simulink model "boithitiko"  (Simulink 5.0)
settings: Solver=FixedStepDiscrete  StartTime=0.0  StopTime=inf  RelTol=1e-3
libraries: dspquant2 x1, dspbuff3 x1
CloseFcn:
  | rtwprivate ssgencode ModelCloseRequest boithitiko
settings Model: LastModifiedBy=efst  RTWOptions="-aEnforceIntegerDowncast=1 -aExtMode=0 -aExtModeTesting=0 -aFoldNonRolledExpr=1 -aForceParamTrailComments=0 -aGenerateComments=1 -aGenerateReport=0 -aIgnoreCustomStorageClasses=1 -aIncDataTypeInIds=0 -aIncHierarchyInIds=0 -aInlineInvariantSignals=0 -aInlinedPrmAccess=\"Literals\" -aLocalBlockOutputs=1 -aLogVarNameModifier=\"rt_\" -aMaxRTWIdLen=31 -aPrefixModelToSubsysFcnNames=1 -aRTWVerbose=1 -aRollThreshold=5 -aShowEliminatedStatements=0"

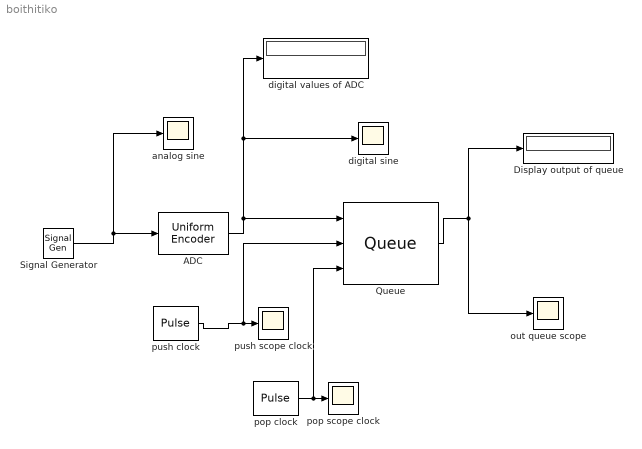
== system boithitiko ==
  ADC : dspquant2/Uniform Encoder  peak=1  bits=8  otype=Unsigned integer
  Display output of queue : Display
  Queue : dspbuff3/Queue  depth=3  trigger=Rising edge  overflow=Dynamic reallocation  pes=Warning  eso=off  fso=off  nso=off  clr=off  clrOutport=off
  Signal Generator : SignalGenerator  Frequency=1000
  analog sine : Scope
      settings: YMin=-1  YMax=1
  digital sine : Scope
      settings: TimeRange=0.001  YMin=0  YMax=275
  digital values of ADC : Display
  out queue scope : Scope
      settings: TimeRange=0.01  YMin=0  YMax=275  SaveName=ScopeData5
  "pop clock " : DiscretePulseGenerator  PulseType=Time based  Period=10^(-4)  PulseWidth=50  PhaseDelay=(10^(-6))/4
  pop scope clock : Scope
      settings: SaveName=ScopeData3
  push clock : DiscretePulseGenerator  PulseType=Time based  Period=10^(-4)  PulseWidth=50
  push scope clock : Scope
      settings: SaveName=ScopeData2
  wires:
  Signal Generator/1 -> analog sine/1, ADC/1
  ADC/1 -> Queue/1, digital values of ADC/1, digital sine/1
  push clock/1 -> push scope clock/1, Queue/2
  "pop clock "/1 -> pop scope clock/1, Queue/3
  Queue/1 -> Display output of queue/1, out queue scope/1
